simulink model "lab2S"  (R2014b)
settings: Solver=ode3  StartTime=0.0  StopTime=10.0  FixedStep=dt  MaxStep=dt  RelTol=1e-3
values from neighbouring files (symbols this model uses):
  den = [1, 15, 85, 225, 274, 120]    [lab6.m]
  num = [0, 0, 0, 1, 3, 2]    [lab6.m]
undefined symbols (not defined in the file or in its folder): dt, input
libraries: simulink x1
settings Model: Creator=lq561d  LastModifiedBy=lq561d

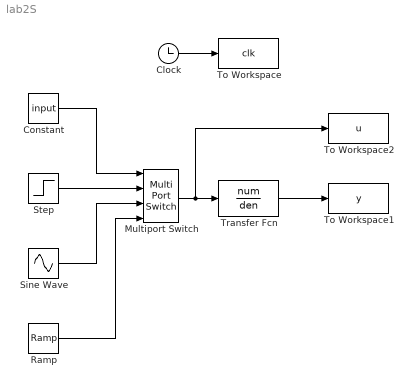
== system lab2S ==
  Clock : Clock
  Constant : Constant  Value=input
  Multiport Switch : MultiPortSwitch
  Ramp : simulink/Sources/Ramp  slope=1  start=0  X0=0
  Sine Wave : Sin  Frequency=100/(2*pi)  SampleTime=dt
  Step : Step  SampleTime=0
  To Workspace : ToWorkspace  VariableName=clk  SampleTime=-1
  To Workspace1 : ToWorkspace  VariableName=y  SampleTime=-1
  To Workspace2 : ToWorkspace  VariableName=u  SampleTime=-1
  Transfer Fcn : TransferFcn  Numerator=num  Denominator=den
  wires:
  Clock/1 -> To Workspace/1
  Transfer Fcn/1 -> To Workspace1/1
  Multiport Switch/1 -> To Workspace2/1, Transfer Fcn/1
  Constant/1 -> Multiport Switch/1
  Step/1 -> Multiport Switch/2
  Sine Wave/1 -> Multiport Switch/3
  Ramp/1 -> Multiport Switch/4
